simulink model "ClosedLoop_encry_2016b"  (R2016b)
settings: Solver=VariableStepAuto  StartTime=0.0  StopTime=2  RelTol=1e-3
undefined symbols (not defined in the file or in its folder): Kha, Kv, wn, zeta
settings Model: Creator=Sarish  LastModifiedBy=Sarish
settings DataIOCC: ReturnWorkspaceOutputs=on
settings SFSimCC: SimUseLocalCustomCode=on
settings RTWCC: RTWUseLocalCustomCode=on

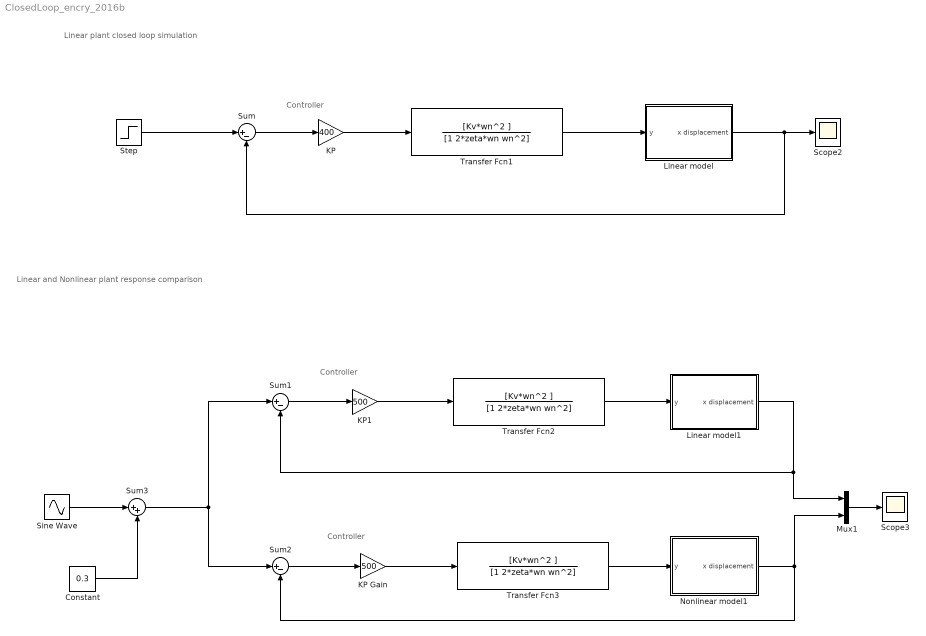
== system ClosedLoop_encry_2016b ==
  note: Linear plant closed loop simulation
  note: Linear and Nonlinear plant response comparison
  note: Controller
  note: Controller
  note: Controller
  Constant : Constant  Value=0.3
  KP : Gain  Gain=400
  KP Gain : Gain  Gain=500
  KP1 : Gain  Gain=500
  Linear model : Subsystem
  Linear model1 : Subsystem
  Mux1 : Mux  Inputs=2
  Nonlinear model1 : Subsystem
      mask help: Simulink:masks:GenSFuncDesc_MD
      mask Help: eval('feval(''rtwprivate'',''rtwhelpview'',''rtw_sfcn_block'')');
  Scope2 : Scope
  Scope3 : Scope
  Sine Wave : Sin  Amplitude=0.15  Frequency=12.57  VectorParams1D=off
  Step : Step  Time=0  Before=0.3  After=0.45  SampleTime=0
  Sum : Sum  Inputs=|+-
  Sum1 : Sum  Inputs=|+-
  Sum2 : Sum  Inputs=|+-
  Sum3 : Sum  Inputs=|++
  Transfer Fcn1 : TransferFcn  Numerator=[Kv*wn^2 ]  Denominator=[1 2*zeta*wn wn^2]
  Transfer Fcn2 : TransferFcn  Numerator=[Kv*wn^2 ]  Denominator=[1 2*zeta*wn wn^2]
  Transfer Fcn3 : TransferFcn  Numerator=[Kv*wn^2 ]  Denominator=[1 2*zeta*wn wn^2]
  wires:
  Sine Wave/1 -> Sum3/1
  Constant/1 -> Sum3/2
  Linear model1/1(x displacement) -> Mux1/1, Sum1/2
  Transfer Fcn1/1 -> Linear model/1(y)
  Sum1/1 -> KP1/1
  Mux1/1 -> Scope3/1
  Sum3/1 -> Sum1/1, Sum2/1
  Nonlinear model1/1(x displacement) -> Sum2/2, Mux1/2
  KP1/1 -> Transfer Fcn2/1
  Sum2/1 -> KP Gain/1
  Step/1 -> Sum/1
  KP Gain/1 -> Transfer Fcn3/1
  KP/1 -> Transfer Fcn1/1
  Sum/1 -> KP/1
  Transfer Fcn2/1 -> Linear model1/1(y)
  Linear model/1(x displacement) -> Sum/2, Scope2/1
  Transfer Fcn3/1 -> Nonlinear model1/1(y)

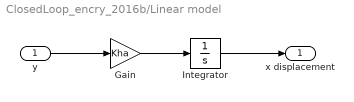
== system ClosedLoop_encry_2016b/Linear model ==
  y : Inport
  Gain : Gain  Gain=Kha
  Integrator : Integrator  InitialCondition=0.3
  x displacement : Outport
  wires:
  y/1 -> Gain/1
  Gain/1 -> Integrator/1
  Integrator/1 -> x displacement/1

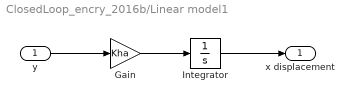
== system ClosedLoop_encry_2016b/Linear model1 ==
  y : Inport
  Gain : Gain  Gain=Kha
  Integrator : Integrator  InitialCondition=0.3
  x displacement : Outport
  wires:
  y/1 -> Gain/1
  Gain/1 -> Integrator/1
  Integrator/1 -> x displacement/1

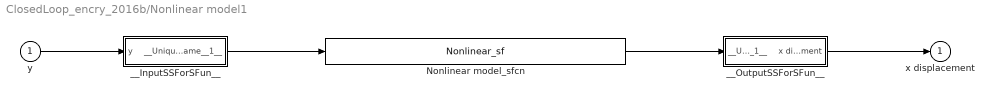
== system ClosedLoop_encry_2016b/Nonlinear model1 ==
  y : Inport
  Nonlinear model_sfcn : S-Function  FunctionName=Nonlinear_sf  SFunctionModules=""  SFunctionDeploymentMode=off  EnableBusSupport=off  mask{rtw_sf_name=Nonlinear_sf, showVar=off}
      mask prompts: rtw_sf_name "Simulink:masks:GenSFuncName_MP"; showVar "Simulink:masks:GenSFuncShowModuleList_MP"
      mask help: Simulink:masks:GenSFuncDesc_MD
      mask init:
      | displist = '';
      | if ~strcmp(get_param(gcb, 'FunctionName'), rtw_sf_name);
      |   set_param(gcb, 'FunctionName', rtw_sf_name);
      | end
      | % Check if we are generating code
      | rtw_mode = false;
      | if strcmpi(get_param(bdroot(gcb),'SimulationStatus'),'Initializing')
      | 	rtw_mode = strcmpi(get_param(bdroot(gcb),'BuildingRTWCode'),'on') && ...
      | 		~strcmpi(get_param(bdroot(gcb),'TargetStyle'),'SimulationTarget');
      | end
      | if showVar || rtw_mode
      | 	if exist('rtwsfunc') == 2 | exist('rtwsfunc') == 6
      | 		tmplist = rtwsfunc(rtw_sf_name,gcb);
      | 		tmplist = DAStudio.message('Simulink:masks:GenSFuncListOfModules_IC', tmplist);
      | 	elseif showVar
      | 		tmplist1 = DAStudio.message('Simulink:masks:GenSFuncListOfModules_IC', '');
      |         tmplist2 = DAStudio.message('Simulink:masks:GenSFuncNotLicensed_IC');
      |         tmplist = [tmplist1 tmplist2];
      |  	end
      | end
      | if showVar
      |   displist = tmplist;
      | end
      settings: CopyFcn=|
      | if ~strcmp(get_param(gcb,'Linkstatus'),'none') && ...
      | ~strcmp(get_param(gcb,'Linkstatus'),'implicit')
      |   set_param(gcb,'LinkStatus','none');
      | end
      mask Help: eval('feval(''rtwprivate'',''rtwhelpview'',''rtw_sfcn_block'')');
      mask Display:
      | port_label('input',1,'y');
      | port_label('output',1,'x displacement');
  __InputSSForSFun__ : Subsystem
  __OutputSSForSFun__ : Subsystem
  x displacement : Outport
  wires:
  __OutputSSForSFun__/1(x displacement) -> x displacement/1
  Nonlinear model_sfcn/1 -> __OutputSSForSFun__/1(__UniqueInportName__1__)
  __InputSSForSFun__/1(__UniqueOutportName__1__) -> Nonlinear model_sfcn/1
  y/1 -> __InputSSForSFun__/1(y)

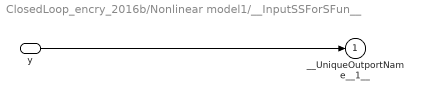
== system ClosedLoop_encry_2016b/Nonlinear model1/__InputSSForSFun__ ==
  y : Inport
  __UniqueOutportName__1__ : Outport
  wires:
  y/1 -> __UniqueOutportName__1__/1

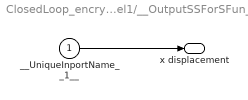
== system ClosedLoop_encry_2016b/Nonlinear model1/__OutputSSForSFun__ ==
  __UniqueInportName__1__ : Inport
  x displacement : Outport
  wires:
  __UniqueInportName__1__/1 -> x displacement/1
